simulink model "Washing_Machine_stateflow"  (R2024b)
settings: Solver=VariableStepAuto  StartTime=0.0  StopTime=inf  RelTol=1e-3
settings Model: Creator=sudee  LastModifiedBy=sudee

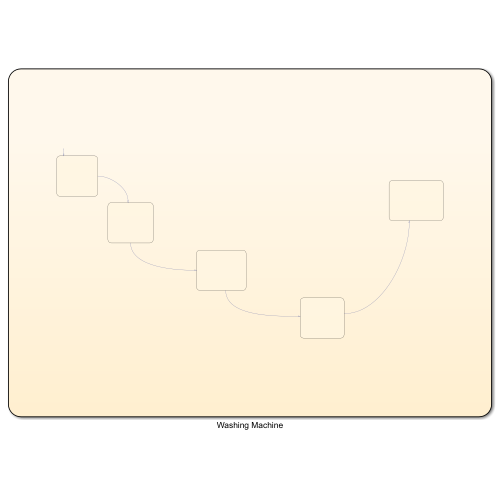
[thumbnail: Simulink's stored preview of the top-level diagram]
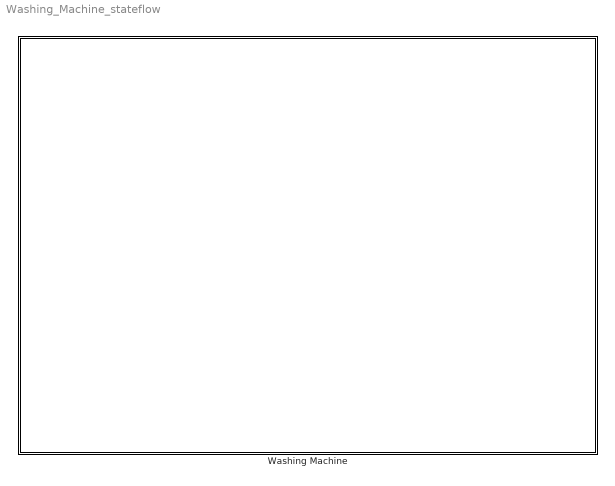
== system Washing_Machine_stateflow ==
  Washing Machine : Stateflow chart  TreatAsAtomicUnit=on

== stateflow chart Washing_Machine_stateflow/Washing Machine ==
  state Fill
    entry:
    disp('Filling water...');
    during:
    fill_time = fill_time + 1;
    exit:
    if fill_time >= Fill_Duration
    disp('Filling Complete.');
    end
    ;
  state Done
    entry:
    disp('Cycle Complete. Washing Done.');
  state Wash
    entry:
    disp('Washing...');
    during:
    wash_time = wash_time + 1;
    exit:
    if wash_time >= Wash_Duration
    disp('Washing Complete.');
    end
  state Rinse
    entry:
    disp('Rinsing...');
    during:
    rinse_time = rinse_time + 1;
    exit:
    if rinse_time >= Rinse_Duration
    disp('Rinsing Complete.');
    end
  state Spin
    entry:
    disp('Spinning...');
    during:
    spin_time = spin_time + 1;
    exit:
    if spin_time >= Spin_Duration
    disp('Spinning Complete.');
    end
  (default) -> Fill
  Fill -> Wash : [after(30, sec)]
  Spin -> Done : [after(40, sec)]
  Wash -> Rinse : [after(40, sec)]
  Rinse -> Spin : [after(40, sec)]
  data: wash_time local =10; spin_time local =10; rinse_time local =10; fill_time local =10; Fill_Duration local double; Rinse_Duration local double; Spin_Duration local double; Wash_Duration local double
